simulink model "danxiangbanboqiaoshizhengliu"  (Simulink 7.3)
settings: Solver=ode15s  StartTime=0.0  StopTime=10  RelTol=1e-3
libraries: powerlib x9, powerlib_extras x3
settings Model: Creator=Administrator  LastModifiedBy=Administrator

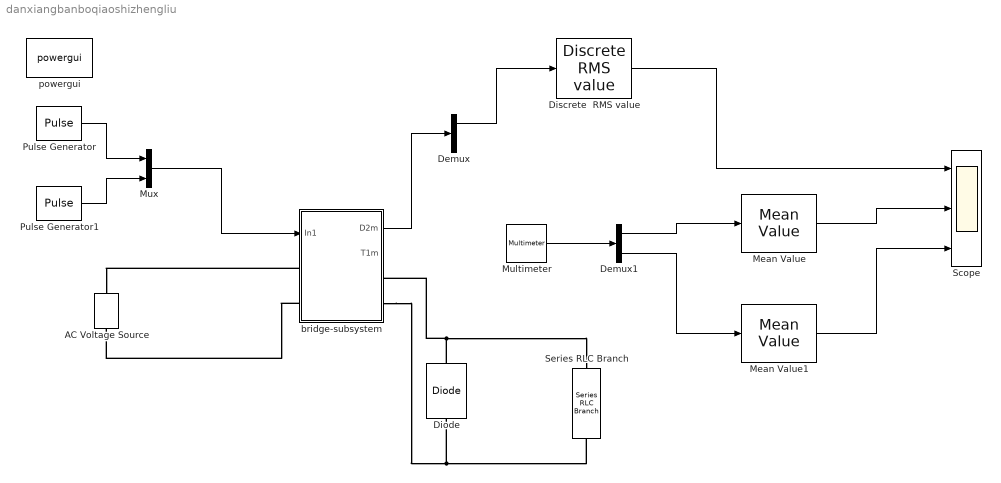
== system danxiangbanboqiaoshizhengliu ==
  AC Voltage Source : powerlib/Electrical Sources/AC Voltage Source  DialogController=POWERSYS.PowerSysDialog  SystemSampleTime=-1  Amplitude=220  Phase=0  Frequency=50  SampleTime=0  Measurements=Voltage
  Demux : Demux  Outputs=2
  Demux1 : Demux  Outputs=2
  Diode : powerlib/Power Electronics/Diode  DialogController=POWERSYS.PowerSysDialog  SystemSampleTime=-1  Ron=0.001  Lon=0  Vf=0.8  IC=0  UseSnubber=off  Rs=500  Cs=250e-9  Measurements=off
  Discrete  RMS value : powerlib_extras/Discrete Measurements/Discrete  RMS value  DialogController=POWERSYS.PowerSysDialog  SystemSampleTime=-1  Freq=60  Mag_Init=0  Ts=50e-6
  Mean Value : powerlib_extras/Measurements/Mean Value  DialogController=POWERSYS.PowerSysDialog  SystemSampleTime=-1  Period=1/60
  Mean Value1 : powerlib_extras/Measurements/Mean Value  DialogController=POWERSYS.PowerSysDialog  SystemSampleTime=-1  Period=1/60
  Multimeter : powerlib/Measurements/Multimeter  SystemSampleTime=-1  PhasorSimulation=off  OutputType=Complex  sel=[1 3]  L=3  Gain=[1 1]  yselected={'Ub: Series RLC Branch','Ib: Series RLC Branch'};  PSBOutputType=1  PSBequivalent=0  AxesSetting=[0,0.1,-100,100]  Display=0  SavedBlockNames=-11
  Mux : Mux  Inputs=2
  Pulse Generator : DiscretePulseGenerator  PulseType=Time based  Amplitude=1  Period=10  PulseWidth=5  PhaseDelay=0.00167  SampleTime=1
  Pulse Generator1 : DiscretePulseGenerator  PulseType=Time based  Amplitude=1  Period=10  PulseWidth=10  PhaseDelay=0.00167*2  SampleTime=1
  Scope : Scope  NumInputPorts=3
      settings: YMin=0~-2.5~-0.25  YMax=60000~42.5~3.5
  Series RLC Branch : powerlib/Elements/Series RLC Branch  DialogController=POWERSYS.PowerSysDialog  PhysicalDomain=powersysdomain  SubClassName=unknown  LeftPortType=p1  RightPortType=p1  LConnTagsString=__new0  RConnTagsString=__new0  BranchType=RL  Resistance=10  Inductance=1  SetiL0=off  InitialCurrent=0  Capacitance=1e-6  Setx0=off  InitialVoltage=0  Measurements=Branch voltage and current
  bridge-subsystem : Subsystem
  powergui : powerlib/powergui  Priority=1  SystemSampleTime=-1  SimulationMode=Continuous  SampleTime=50e-6  frequency=60  SPID=off  DisableSnubberDevices=off  DisableRonSwitches=off  DisableVfSwitches=off  SwTol=0  Interpol=off  frequencyindice=50  echomessages=off  HookPort=off  DisplayEquations=off  FunctionMessages=off  EnableUseOfTLC=off  x0status=blocks  RestoreLinks=warning  Frange=[0:2:500]  Ylog=off  Xlog=on  ShowGrid=off  save=off  variable=ZData  ZoomFFT=on  StartTime=0.0  cycles=1  DisplayStyle=1  fundamental=60  FreqAxis=off  MaxFrequency=1000  frequencyindicesteady=1  RmsSteady=1  display=off  Ts=0  methode=off
  wires:
  Pulse Generator/1 -> Mux/1
  Pulse Generator1/1 -> Mux/2
  Demux/1 -> Discrete  RMS value/1
  bridge-subsystem/1(D2m) -> Demux/1
  Multimeter/1 -> Demux1/1
  Discrete  RMS value/1 -> Scope/1
  Mean Value1/1 -> Scope/3
  Mean Value/1 -> Scope/2
  Demux1/1 -> Mean Value/1
  Demux1/2 -> Mean Value1/1
  Mux/1 -> bridge-subsystem/1(In1)
  connections:
  bridge-subsystem/RConn1 -- Diode/RConn1 -- Series RLC Branch/LConn1
  bridge-subsystem/RConn2 -- Series RLC Branch/RConn1 -- Diode/LConn1
  bridge-subsystem/LConn2 -- AC Voltage Source/LConn1
  bridge-subsystem/LConn1 -- AC Voltage Source/RConn1

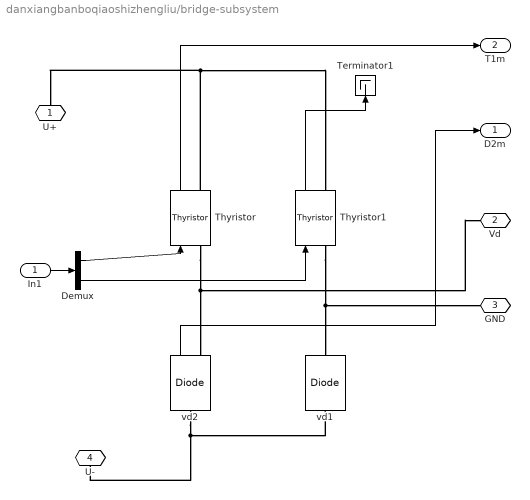
== system danxiangbanboqiaoshizhengliu/bridge-subsystem ==
  In1 : Inport
  Demux : Demux  Outputs=2
  Terminator1 : Terminator
  Thyristor : powerlib/Power Electronics/Thyristor  DialogController=POWERSYS.PowerSysDialog  SystemSampleTime=-1  Ron=0.001  Lon=0  Vf=0.8  IC=0  Rs=500  Cs=250e-9  Measurements=on
  Thyristor1 : powerlib/Power Electronics/Thyristor  DialogController=POWERSYS.PowerSysDialog  SystemSampleTime=-1  Ron=0.001  Lon=0  Vf=0.8  IC=0  Rs=500  Cs=250e-9  Measurements=on
  vd1 : powerlib/Power Electronics/Diode  DialogController=POWERSYS.PowerSysDialog  SystemSampleTime=-1  Ron=0.001  Lon=0  Vf=0.8  IC=0  UseSnubber=off  Rs=500  Cs=250e-9  Measurements=off
  vd2 : powerlib/Power Electronics/Diode  DialogController=POWERSYS.PowerSysDialog  SystemSampleTime=-1  Ron=0.001  Lon=0  Vf=0.8  IC=0  UseSnubber=off  Rs=500  Cs=250e-9  Measurements=on
  U+ : PMIOPort  Port=1  Side=Left
  Vd : PMIOPort  Port=2  Side=Right
  GND : PMIOPort  Port=3  Side=Right
  U- : PMIOPort  Port=4  Side=Left
  D2m : Outport  OutDataType=fixdt(1, 16)  OutScaling=2^0
  T1m : Outport  Port=2  OutDataType=fixdt(1, 16)  OutScaling=2^0
  wires:
  Demux/1 -> Thyristor/1
  Demux/2 -> Thyristor1/1
  In1/1 -> Demux/1
  Thyristor1/1 -> Terminator1/1
  Thyristor/1 -> T1m/1
  vd2/1 -> D2m/1
  connections:
  U-/RConn1 -- vd2/LConn1 -- vd1/LConn1
  Vd/RConn1 -- Thyristor/LConn1 -- vd2/RConn1
  Thyristor1/LConn1 -- vd1/RConn1 -- GND/RConn1
  Thyristor/RConn1 -- Thyristor1/RConn1 -- U+/RConn1
